simulink model "PendulumRCSPlantWPsi"  (R2018b)
settings: Solver=VariableStepAuto  StartTime=0.0  StopTime=20  RelTol=1e-9
values from neighbouring files (symbols this model uses):
  k_tor = 1    [GenPendulumParams.m]
  L = 3    [GenPendulumParams.m]
  M = 1.79    [GenPendulumParams.m]
  rho_tor = 0.5    [GenPendulumParams.m]
libraries: sharedutil x1, shared6dof x1, vrlib x1
settings Model: OrderedModelArguments=off  Creator=mendicantbias  LastModifiedBy=mendicantbias
settings ModelReferenceCC: ModelReferenceNumInstancesAllowed=Single

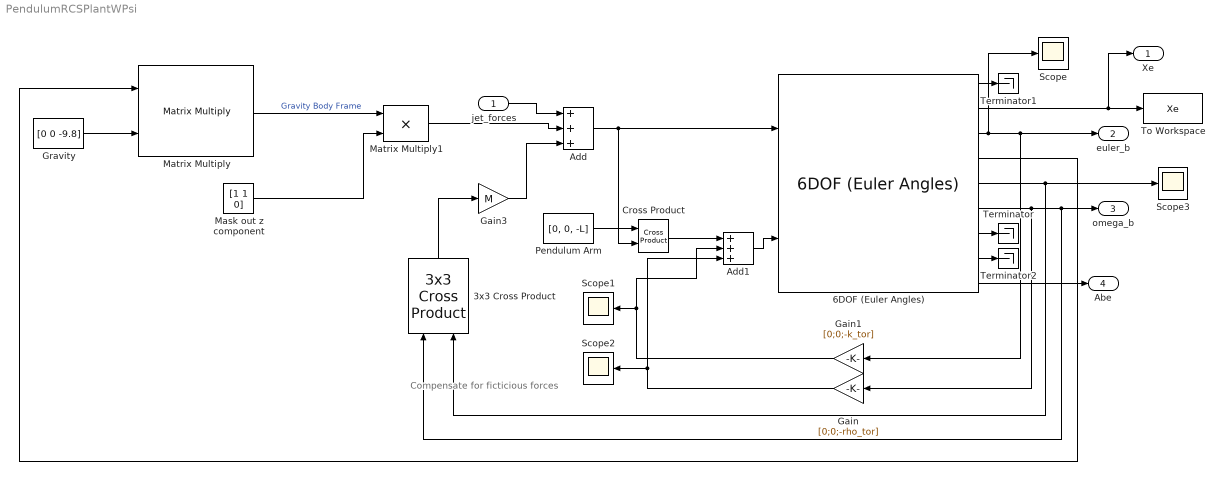
== system PendulumRCSPlantWPsi ==
  note: Compensate for ficticious forces
  jet_forces : Inport  PortDimensions=3
  3x3 Cross Product : sharedutil/3x3 Cross Product  aMode=aMode
      settings: SourceProductBaseCode=AE
  6DOF (Euler Angles) : shared6dof/6DOF (Euler Angles)  units=Metric (MKS)  mtype=Fixed  rep=Euler Angles  xme_0=[0 0 -L]  Vm_0=[0 0 0]  eul_0=[0 0 0]  pm_0=w0  mass_0=M  mass_e=0.5  mass_f=2.0  inertia=I  inertia_e=eye(3)  inertia_f=2*eye(3)  k_quat=1.0  vre_flag=on  abi_flag=on  aMode=0  xme_statename=''  Vm_statename=''  eul_statename=''  quat_statename=''  pm_statename=''  mass_statename=''
      settings: SourceProductBaseCode=AE
  Add : Sum  Inputs=+++
  Add1 : Sum  Inputs=+++
  Cross Product : vrlib/Utilities/Cross Product
      settings: SourceProductBaseCode=VR
  Gain : Gain  Gain=[0;0;-rho_tor]
  Gain1 : Gain  Gain=[0;0;-k_tor]
  Gain3 : Gain  Gain=M
  Gravity : Constant  Value=[0 0 -9.8]
  Mask out z component : Constant  Value=[1 1 0]
  Matrix Multiply : Product  Multiplication=Matrix(*)
  Matrix Multiply1 : Product
  Pendulum Arm : Constant  Value=[0, 0, -L]
  Scope{,1..3} (4 alike) : Scope
  Terminator : Terminator
  Terminator1 : Terminator
  Terminator2 : Terminator
  To Workspace : ToWorkspace  VariableName=Xe  SaveFormat=Timeseries  SampleTime=-1
  Xe : Outport
  euler_b : Outport  Port=2
  omega_b : Outport  Port=3
  Abe : Outport  Port=4
  wires:
  Matrix Multiply/1 -> Matrix Multiply1/1  "Gravity Body Frame"
  Gravity/1 -> Matrix Multiply/2
  6DOF (Euler Angles)/4 -> Matrix Multiply/1
  Add/1 -> 6DOF (Euler Angles)/1, Cross Product/2
  Pendulum Arm/1 -> Cross Product/1
  6DOF (Euler Angles)/6 -> Gain/1, omega_b/1, 3x3 Cross Product/1
  6DOF (Euler Angles)/5 -> 3x3 Cross Product/2, Scope3/1
  Mask out z component/1 -> Matrix Multiply1/2
  Matrix Multiply1/1 -> Add/2
  3x3 Cross Product/1 -> Gain3/1
  Gain3/1 -> Add/3
  6DOF (Euler Angles)/7 -> Terminator/1
  6DOF (Euler Angles)/1 -> Terminator1/1
  6DOF (Euler Angles)/8 -> Terminator2/1
  6DOF (Euler Angles)/2 -> Xe/1, To Workspace/1
  6DOF (Euler Angles)/3 -> euler_b/1, Gain1/1, Scope/1
  6DOF (Euler Angles)/9 -> Abe/1
  Gain1/1 -> Add1/2, Scope1/1
  Gain/1 -> Scope2/1, Add1/3
  Cross Product/1 -> Add1/1
  Add1/1 -> 6DOF (Euler Angles)/2
  jet_forces/1 -> Add/1
